simulink model "ps10"  (R2020b)
settings: Solver=VariableStepAuto  StartTime=0.0  StopTime=10.0  RelTol=1e-3
libraries: simulink x3, fl_lib x1
settings Model: Creator=prana  LastModifiedBy=prana

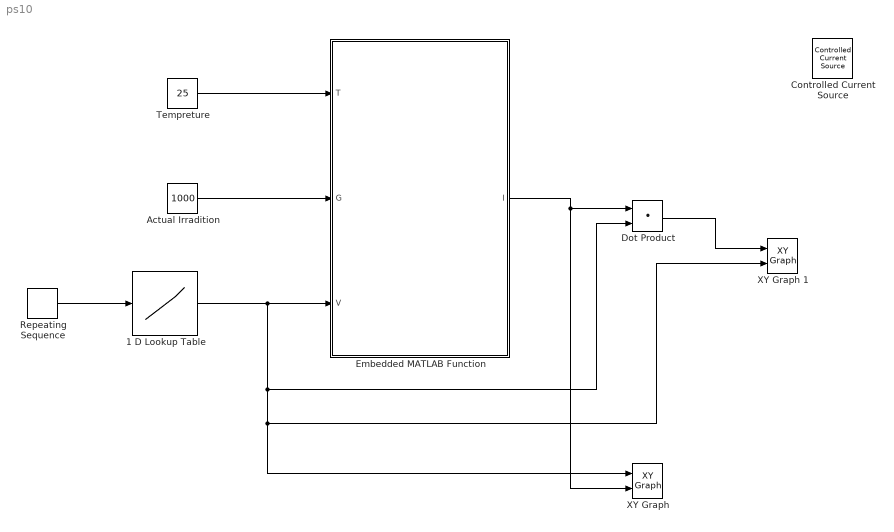
== system ps10 ==
  1 D Lookup Table : Lookup_n-D  NumberOfTableDimensions=1  BreakpointsForDimension1=[-5:5]  Table=tanh([-5:5])  InternalRulePriority=Speed  RndMeth=Simplest  InputSameDT=on
  Actual Irradition : Constant  Value=1000
  Controlled Current Source : fl_lib/Electrical/Electrical Sources/Controlled Current Source
  "Dot Product " : DotProduct  InputSameDT=on  OutDataTypeStr=Inherit: Inherit via internal rule
  Embedded MATLAB Function : MATLAB Function  TreatAsAtomicUnit=on
  "Repeating Sequence " : simulink/Sources/Repeating Sequence  rep_seq_t=[0 2]  rep_seq_y=[0 2]
  Tempreture : Constant  Value=25
  XY Graph : simulink/Sinks/XY Graph  xmin=-1  xmax=1  ymin=-1  ymax=1  st=-1
  XY Graph 1 : simulink/Sinks/XY Graph  xmin=-1  xmax=1  ymin=-1  ymax=1  st=-1
  wires:
  "Repeating Sequence "/1 -> 1 D Lookup Table/1
  Embedded MATLAB Function/1(I) -> XY Graph/2, "Dot Product "/1
  Tempreture/1 -> Embedded MATLAB Function/1(T)
  Actual Irradition/1 -> Embedded MATLAB Function/2(G)
  "Dot Product "/1 -> XY Graph 1/1
  1 D Lookup Table/1 -> XY Graph 1/2, XY Graph/1, "Dot Product "/2, Embedded MATLAB Function/3(V)

== matlab function ps10/Embedded MATLAB Function ==
  data: T input; I output; G input; V input
function I= fcn(T, G, V)
clc;
K = 1.38065e-23;   %boltzman constatnt
q = 1.602e-19      %charge of electron
Iscn = 8.21;       %nominal SC current
Vocn = 32.9;       %nominal OC voltage
Kv = -0.123;       %tempreture voltage const
Ki = 0.0032;       %tempreture current const
Ns = 54;           %no of series connected cells
T = T+273;        %operating temp
Tn = 25+273;       %nominal temp
Gn = 1050;         %nominal Irradiance
a = 1.3;           %diode ideality constant
Eg = 1.12;         %band gap of SI @25deg
%G = 1000;          %actual irradition
Rs = 0.221;
Rp = 415.405;
I=0;
Vtn = Ns*(K*Tn/q);

Ion = Iscn/((exp(Vocn/(a*Vtn)))-1);

Io_part =  ((q*Eg/(a*K))*((1/Tn)-(1/T)));
Io = Ion*((Tn/T)^3)*exp(Io_part);
Ipvn = Iscn;

Ipv = (Ipvn + Ki*(T-Tn))*(G/Gn);

Vt = Ns*(K*T/q);
I_part = Io*(exp((V+(I*Rs))/(Vt*a))-1) + ((V+(Rs*I))/Rp);

I= Ipv - I_part;
